simulink model "test1"  (R2024a)
settings: Solver=FixedStepAuto  StartTime=0.0  StopTime=5  FixedStep=0.0001  RelTol=1e-3  EnableMultiTasking=on
undefined symbols (not defined in the file or in its folder): d_x_0, d_y_0, d_z_0, g, Jx, Jy, Jz, m, omegabx_0, omegaby_0, omegabz_0, phi_0, psi_0, theta_0, x_0, y_0, z_0
settings Model: Creator=Administrator  LastModifiedBy=Zhenkai
settings SolverCC: AlgebraicLoopSolver=TrustRegion
settings DataIOCC: ReturnWorkspaceOutputs=off
settings OptimizationCC: LifeSpan=inf
settings DebuggingCC: UnconnectedInputMsg=warning  UnconnectedOutputMsg=warning  UnconnectedLineMsg=warning  SFUnexpectedBacktrackingDiag=warning  SFNoUnconditionalDefaultTransitionDiag=warning  ArithmeticOperatorsInVariantConditions=warning
settings ModelReferenceCC: EnableRefExpFcnMdlSchedulingChecks=on
settings SFSimCC: SimUseLocalCustomCode=off  CustomCodeUndefinedFunction=UseInterfaceOnly
settings RTWCC: RTWUseLocalCustomCode=off  GPUComputeCapability=3.5
settings CodeAppCC: StateflowObjectComments=on
settings GRTTargetCC: TargetLangStandard=C89/C90 (ANSI)
settings ConfigComp: CovMetricSettings=dw  CovSaveCumulativeToWorkspaceVar=on  CovSaveSingleToWorkspaceVar=on  CovExternalEMLEnable=off

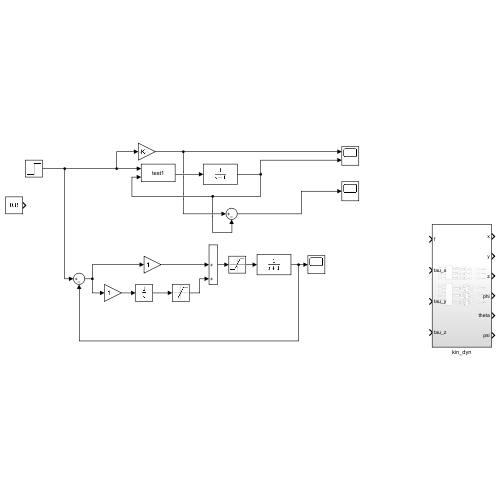
[thumbnail: Simulink's stored preview of the top-level diagram]
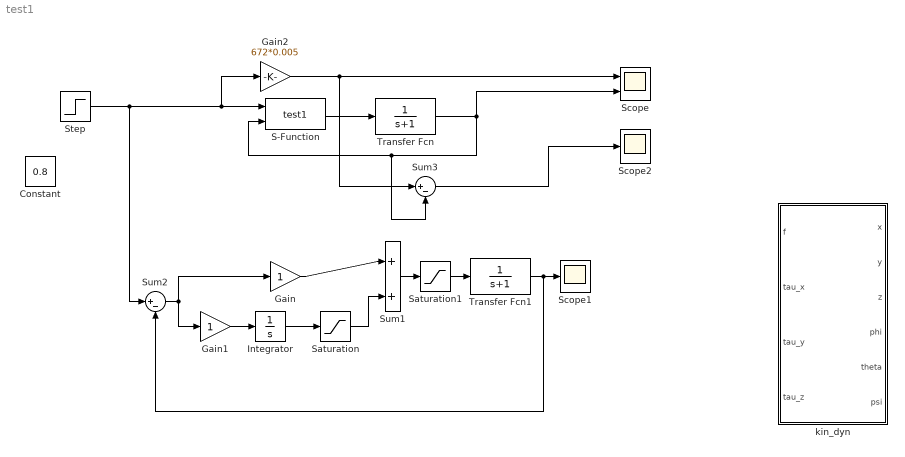
== system test1 ==
  Constant : Constant  Value=0.8
  Gain : Gain
  Gain1 : Gain
  Gain2 : Gain  Gain=672*0.005
  Integrator : Integrator
  S-Function : S-Function  FunctionName=test1  SFunctionDeploymentMode=off  EnableBusSupport=off
  Saturation : Saturate  UpperLimit=70  LowerLimit=-70
  Saturation1 : Saturate  UpperLimit=70  LowerLimit=-70
  Scope : Scope  NumInputPorts=2
  Scope1 : Scope
  Scope2 : Scope
  Step : Step  SampleTime=0
  Sum1 : Sum  Inputs=|++
  Sum2 : Sum  Inputs=|+-
  Sum3 : Sum  Inputs=|+-
  Transfer Fcn : TransferFcn  Denominator=[1 1]
  Transfer Fcn1 : TransferFcn  Denominator=[1 1]
  kin_dyn : Subsystem
  wires:
  Transfer Fcn/1 -> S-Function/2, Sum3/2, Scope/2
  Sum1/1 -> Saturation1/1
  Integrator/1 -> Saturation/1
  Gain1/1 -> Integrator/1
  Gain/1 -> Sum1/1
  Saturation/1 -> Sum1/2
  Saturation1/1 -> Transfer Fcn1/1
  Transfer Fcn1/1 -> Sum2/2, Scope1/1
  Sum2/1 -> Gain1/1, Gain/1
  S-Function/1 -> Transfer Fcn/1
  Step/1 -> Gain2/1, S-Function/1, Sum2/1
  Gain2/1 -> Sum3/1, Scope/1
  Sum3/1 -> Scope2/1

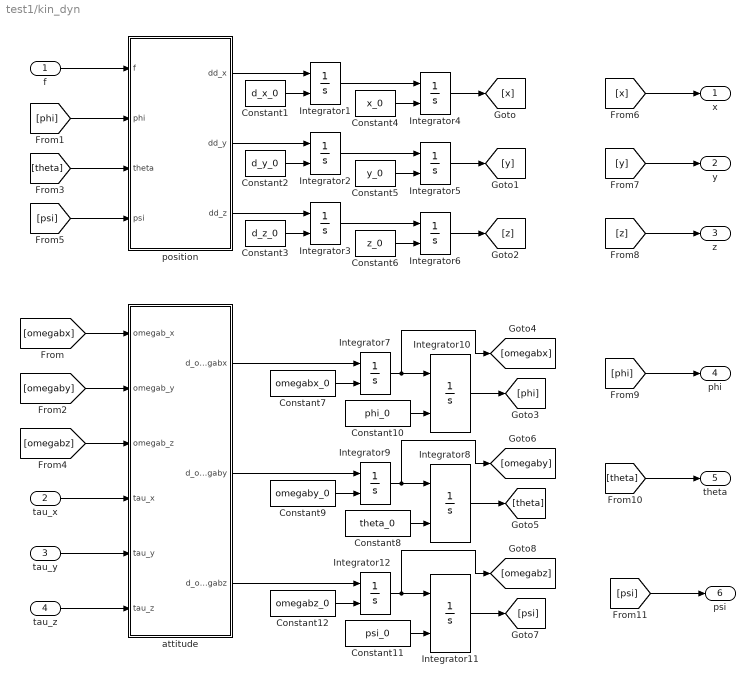
== system test1/kin_dyn ==
  f : Inport
  tau_x : Inport  Port=2
  tau_y : Inport  Port=3
  tau_z : Inport  Port=4
  Constant1 : Constant  Value=d_x_0
  Constant10 : Constant  Value=phi_0
  Constant11 : Constant  Value=psi_0
  Constant12 : Constant  Value=omegabz_0
  Constant2 : Constant  Value=d_y_0
  Constant3 : Constant  Value=d_z_0
  Constant4 : Constant  Value=x_0
  Constant5 : Constant  Value=y_0
  Constant6 : Constant  Value=z_0
  Constant7 : Constant  Value=omegabx_0
  Constant8 : Constant  Value=theta_0
  Constant9 : Constant  Value=omegaby_0
  Integrator{1..12} (12 alike) : Integrator  InitialConditionSource=external
  attitude : Subsystem
  position : Subsystem
  x : Outport
  y : Outport  Port=2
  z : Outport  Port=3
  phi : Outport  Port=4
  theta : Outport  Port=5
  psi : Outport  Port=6
  wires:
  Integrator6/1 -> [z]
  Constant2/1 -> Integrator2/2
  Constant5/1 -> Integrator5/2
  Constant8/1 -> Integrator8/2
  Constant7/1 -> Integrator7/2
  [omegabx] -> attitude/1(omegab_x)
  Integrator2/1 -> Integrator5/1
  [theta] -> theta/1
  Integrator1/1 -> Integrator4/1
  attitude/1(d_omegabx) -> Integrator7/1
  Integrator5/1 -> [y]
  tau_x/1 -> attitude/4(tau_x)
  Integrator7/1 -> [omegabx], Integrator10/1
  tau_y/1 -> attitude/5(tau_y)
  Constant11/1 -> Integrator11/2
  f/1 -> position/1(f)
  attitude/2(d_omegaby) -> Integrator9/1
  [theta] -> position/3(theta)
  Integrator11/1 -> [psi]
  [psi] -> psi/1
  Integrator9/1 -> [omegaby], Integrator8/1
  Constant9/1 -> Integrator9/2
  attitude/3(d_omegabz) -> Integrator12/1
  Integrator12/1 -> [omegabz], Integrator11/1
  position/2(dd_y) -> Integrator2/1
  [x] -> x/1
  Constant10/1 -> Integrator10/2
  [phi] -> position/2(phi)
  Integrator4/1 -> [x]
  [y] -> y/1
  [phi] -> phi/1
  Constant4/1 -> Integrator4/2
  Constant12/1 -> Integrator12/2
  Constant6/1 -> Integrator6/2
  Integrator8/1 -> [theta]
  Constant1/1 -> Integrator1/2
  tau_z/1 -> attitude/6(tau_z)
  [psi] -> position/4(psi)
  Integrator3/1 -> Integrator6/1
  Constant3/1 -> Integrator3/2
  position/1(dd_x) -> Integrator1/1
  position/3(dd_z) -> Integrator3/1
  [z] -> z/1
  [omegaby] -> attitude/2(omegab_y)
  Integrator10/1 -> [phi]
  [omegabz] -> attitude/3(omegab_z)

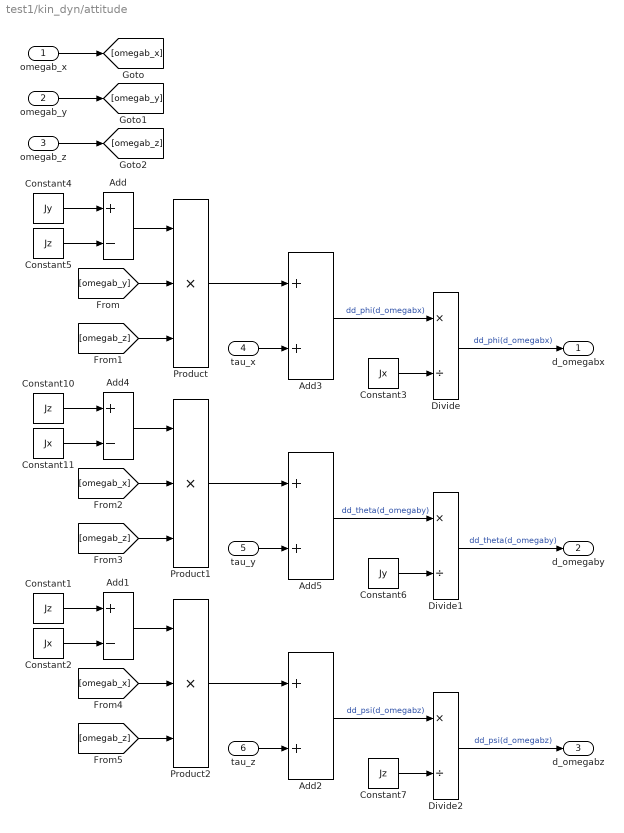
== system test1/kin_dyn/attitude ==
  omegab_x : Inport
  omegab_y : Inport  Port=2
  omegab_z : Inport  Port=3
  tau_x : Inport  Port=4
  tau_y : Inport  Port=5
  tau_z : Inport  Port=6
  Add : Sum  Inputs=+-
  Add1 : Sum  Inputs=+-
  Add2 : Sum
  Add3 : Sum
  Add4 : Sum  Inputs=+-
  Add5 : Sum
  Constant{1,5,7,10} (4 alike) : Constant  Value=Jz
  Constant11 : Constant  Value=Jx
  Constant2 : Constant  Value=Jx
  Constant3 : Constant  Value=Jx
  Constant4 : Constant  Value=Jy
  Constant6 : Constant  Value=Jy
  Divide : Product  Inputs=*/
  Divide1 : Product  Inputs=*/
  Divide2 : Product  Inputs=*/
  Product : Product  Inputs=3
  Product1 : Product  Inputs=3
  Product2 : Product  Inputs=3
  d_omegabx : Outport
  d_omegaby : Outport  Port=2
  d_omegabz : Outport  Port=3
  wires:
  Constant3/1 -> Divide/2
  Constant7/1 -> Divide2/2
  [omegab_z] -> Product/3
  Constant5/1 -> Add/2
  Add/1 -> Product/1
  Constant1/1 -> Add1/1
  Add3/1 -> Divide/1  "dd_phi(d_omegabx)"
  omegab_y/1 -> [omegab_y]
  Add4/1 -> Product1/1
  tau_x/1 -> Add3/2
  Add2/1 -> Divide2/1  "dd_psi(d_omegabz)"
  Divide/1 -> d_omegabx/1  "dd_phi(d_omegabx)"
  Constant4/1 -> Add/1
  omegab_x/1 -> [omegab_x]
  Product/1 -> Add3/1
  omegab_z/1 -> [omegab_z]
  [omegab_x] -> Product2/2
  Divide2/1 -> d_omegabz/1  "dd_psi(d_omegabz)"
  Divide1/1 -> d_omegaby/1  "dd_theta(d_omegaby)"
  [omegab_y] -> Product/2
  Add5/1 -> Divide1/1  "dd_theta(d_omegaby)"
  [omegab_z] -> Product2/3
  [omegab_z] -> Product1/3
  Constant6/1 -> Divide1/2
  tau_z/1 -> Add2/2
  Add1/1 -> Product2/1
  Constant2/1 -> Add1/2
  Product2/1 -> Add2/1
  Constant11/1 -> Add4/2
  tau_y/1 -> Add5/2
  [omegab_x] -> Product1/2
  Constant10/1 -> Add4/1
  Product1/1 -> Add5/1

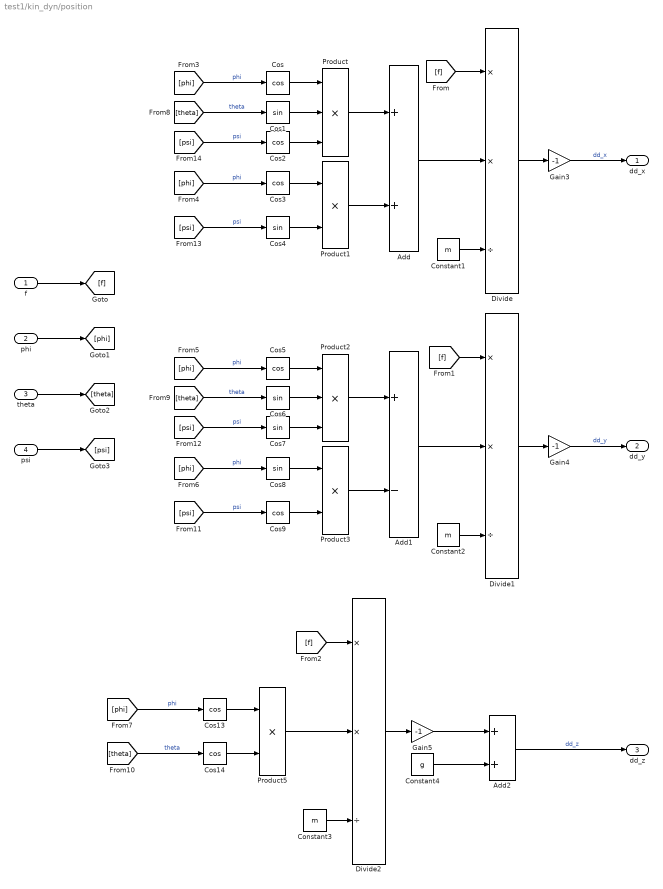
== system test1/kin_dyn/position ==
  f : Inport
  phi : Inport  Port=2
  theta : Inport  Port=3
  psi : Inport  Port=4
  Add : Sum
  Add1 : Sum  Inputs=+-
  Add2 : Sum
  Constant1 : Constant  Value=m
  Constant2 : Constant  Value=m
  Constant3 : Constant  Value=m
  Constant4 : Constant  Value=g
  Cos{,2..3,5,9,13..14} (7 alike) : Trigonometry  Operator=cos
  Cos{1,4,6..8} (5 alike) : Trigonometry
  Divide : Product  Inputs=**/
  Divide1 : Product  Inputs=**/
  Divide2 : Product  Inputs=**/
  Gain3 : Gain  Gain=-1
  Gain4 : Gain  Gain=-1
  Gain5 : Gain  Gain=-1
  Product : Product  Inputs=3
  Product1 : Product
  Product2 : Product  Inputs=3
  Product3 : Product
  Product5 : Product
  dd_x : Outport
  dd_y : Outport  Port=2
  dd_z : Outport  Port=3
  wires:
  Cos/1 -> Product/1
  f/1 -> [f]
  Product/1 -> Add/1
  [f] -> Divide/1
  Add2/1 -> dd_z/1  "dd_z"
  psi/1 -> [psi]
  [phi] -> Cos8/1  "phi"
  Divide/1 -> Gain3/1
  Cos5/1 -> Product2/1
  phi/1 -> [phi]
  [psi] -> Cos9/1  "psi"
  Gain4/1 -> dd_y/1  "dd_y"
  Cos2/1 -> Product/3
  [f] -> Divide2/1
  Add1/1 -> Divide1/2
  Cos1/1 -> Product/2
  Constant2/1 -> Divide1/3
  Constant4/1 -> Add2/2
  Product3/1 -> Add1/2
  Cos6/1 -> Product2/2
  Cos7/1 -> Product2/3
  Cos14/1 -> Product5/2
  Add/1 -> Divide/2
  Divide1/1 -> Gain4/1
  [phi] -> Cos3/1  "phi"
  Cos8/1 -> Product3/1
  Cos9/1 -> Product3/2
  [psi] -> Cos7/1  "psi"
  Divide2/1 -> Gain5/1
  [f] -> Divide1/1
  Product2/1 -> Add1/1
  [phi] -> Cos/1  "phi"
  Cos4/1 -> Product1/2
  Constant3/1 -> Divide2/3
  Product5/1 -> Divide2/2
  Product1/1 -> Add/2
  Cos3/1 -> Product1/1
  [theta] -> Cos6/1  "theta"
  [psi] -> Cos4/1  "psi"
  [psi] -> Cos2/1  "psi"
  Cos13/1 -> Product5/1
  Constant1/1 -> Divide/3
  Gain5/1 -> Add2/1
  Gain3/1 -> dd_x/1  "dd_x"
  [theta] -> Cos14/1  "theta"
  [phi] -> Cos13/1  "phi"
  [phi] -> Cos5/1  "phi"
  theta/1 -> [theta]
  [theta] -> Cos1/1  "theta"
